simulink model "model_with_phases"  (R2018b)
settings: Solver=daessc  StartTime=0.0  StopTime=1  RelTol=1e-3
StopFcn:
  | % fault = 10
  | % location = 200
  | % fault_data
  | % simout=[simout,faults]
  | % simout(:,24) = location;
  | % data = xlsread('E:\testing data\test_data');
  | % data = [data;simout];
  | % xlswrite('E:\testing data\test_data',data);
libraries: powerlib x7, powerlib_meascontrol x2
settings Model: Creator=Edagotti Pavankumar  LastModifiedBy=Edagotti Pavankumar
settings SolverCC: ZeroCrossAlgorithm=Adaptive
settings DebuggingCC: IgnoredZcDiagnostic=none

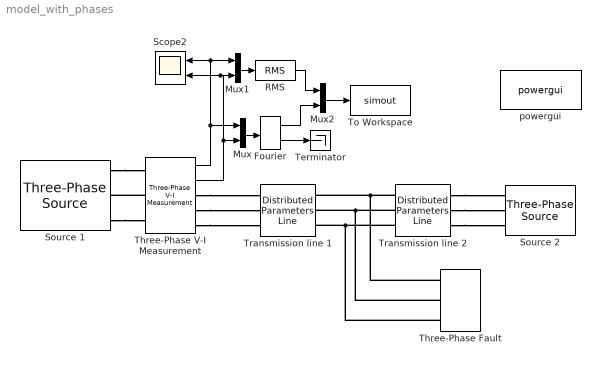
== system model_with_phases ==
  Fourier : powerlib_meascontrol/Measurements/Fourier  Freq=50  n=1  InInit=[0, 0]  Ts=0
      settings: SourceProductName=Simscape Power Systems
  Mux : Mux  Inputs=2
  Mux1 : Mux  Inputs=2
  Mux2 : Mux  Inputs=2
  RMS : powerlib_meascontrol/Measurements/RMS  TrueRMS=on  Freq=50  RMSInit=0  Ts=0
  Scope2 : Scope  NumInputPorts=2
  Source 1 : powerlib/Electrical Sources/Three-Phase Source  InternalConnection=Yg  VoltagePhases=off  Voltage=220e3  PhaseAngle=0  Voltage_phases=[25e3 25e3 25e3]/sqrt(3)  PhaseAngles_phases=[0 -120 +120]  Frequency=50  NonIdealSource=on  SpecifyImpedance=on  Resistance=0.8929  Inductance=16.58e-3  ShortCircuitLevel=100e6  BaseVoltage=220e3  XRratio=7  BusType=swing  Pref=10e3  Qref=0  Prefabc=[10e3, 10e3, 10e3]  Qrefabc=[0, 0, 0]  Qmin=-inf  Qmax=inf
  Source 2 : powerlib/Electrical Sources/Three-Phase Source  InternalConnection=Yg  VoltagePhases=off  Voltage=220e3  PhaseAngle=-40  Voltage_phases=[25e3 25e3 25e3]/sqrt(3)  PhaseAngles_phases=[0 -120 +120]  Frequency=50  NonIdealSource=on  SpecifyImpedance=on  Resistance=0.8929  Inductance=16.58e-3  ShortCircuitLevel=100e6  BaseVoltage=220e3  XRratio=7  BusType=PV  Pref=inf  Qref=0  Prefabc=[10e3, 10e3, 10e3]  Qrefabc=[0, 0, 0]  Qmin=-inf  Qmax=inf
  Terminator : Terminator
  Three-Phase V-I Measurement : powerlib/Measurements/Three-Phase V-I Measurement  VoltageMeasurement=phase-to-ground  SetLabelV=off  LabelV=Vabc  Vpu=on  VpuLL=off  CurrentMeasurement=yes  SetLabelI=off  LabelI=Iabc  Ipu=on  Pbase=100e6  Vbase=220e3  OutputType=Complex  PhasorSimulation=off  PSBequivalent=0
  Three-Phase Fault : powerlib/Elements/Three-Phase Fault  InitialStates=0  FaultA=on  FaultB=off  FaultC=off  GroundFault=on  SwitchTimes=0.5  External=off  SwitchStatus=NaN  FaultResistance=20  GroundResistance=0.001  SnubberResistance=1e6  SnubberCapacitance=inf  Measurements=None
  To Workspace : ToWorkspace  VariableName=simout  SampleTime=-1
      settings: MaxDataPoints=200  Save2DSignal=2-D array (concatenate along first dimension)
  Transmission line 1 : powerlib/Elements/Distributed Parameters Line  Phases=3  Frequency=50  Resistance=[0.0238 0.3885]  Inductance=[0.0009509508 0.0032508989]  Capacitance=[12.74e-9 7.751e-9]  Length=160  x1=[8.85875852267748e-10 256106.737010838 256106.73701084;314.159265358979 314.159265358979 314.159265358979;-0.991239322998321 -0.0183316743636767 -1.58912800115857]  x2=[8.93084897335148e-10 257720.727111479 257720.727111481;314.159265358979 314.159265358979 314.159265358979;-1.00602777839429 -0.045748220316972 -1.61654454711186]  x3=[1.76591819123062e-12 793.390665840204 793.390665840216;314.159265358979 314.159265358979 314.159265358979;-1.42146556624267 -0.176195220133282 -1.74699154692818]  x4=[1.53917367282649e-12 1076.93135796091 1076.93135796091;314.159265358979 314.159265358979 314.159265358979;-0.688414818704923 -0.0783802254355052 -1.6491765522304]  x5=0.000803157247848664  V1=[8.859e-10 2.561e+05 2.561e+05;314.2 314.2 314.2;-0.9912 -0.01833 -1.589]  V2=[8.931e-10 2.577e+05 2.577e+05;314.2 314.2 314.2;-1.006 -0.04575 -1.617]  I1=[1.766e-12 793.4 793.4;314.2 314.2 314.2;-1.421 -0.1762 -1.747]  I2=[1.539e-12 1077 1077;314.2 314.2 314.2;-0.6884 -0.07838 -1.649]  nHarmo=1  Measurements=None
      settings: SourceProductName=Simscape Power Systems
  Transmission line 2 : powerlib/Elements/Distributed Parameters Line  Phases=3  Frequency=50  Resistance=[0.0238 0.3885]  Inductance=[0.0009509508 0.0032508989]  Capacitance=[12.74e-9 7.751e-9]  Length=40  x1=[8.95741011278727e-10 257720.727111479 257720.727111481;314.159265358979 314.159265358979 314.159265358979;-0.814008885135909 0.085470215602079 -1.48532611119281]  x2=[8.89113759047248e-10 256920.332809656 256920.332809659;314.159265358979 314.159265358979 314.159265358979;-0.820988530494618 0.0790008961846263 -1.49179543061027]  x3=[2.24350221076048e-12 798.289373210214 798.289373210219;314.159265358979 314.159265358979 314.159265358979;-2.13671936046073 0.129729677301786 -1.44106664949311]  x4=[9.68167740404967e-13 1084.26106264654 1084.26106264656;314.159265358979 314.159265358979 314.159265358979;0.706934938878884 0.00929096905672002 -1.56150535773818]  x5=0.000200789311962166  V1=[8.957e-10 2.577e+05 2.577e+05;314.2 314.2 314.2;-0.814 0.08547 -1.485]  V2=[8.891e-10 2.569e+05 2.569e+05;314.2 314.2 314.2;-0.821 0.079 -1.492]  I1=[2.244e-12 798.3 798.3;314.2 314.2 314.2;-2.137 0.1297 -1.441]  I2=[9.682e-13 1084 1084;314.2 314.2 314.2;0.7069 0.009291 -1.562]  nHarmo=1  Measurements=None
      settings: SourceProductName=Simscape Power Systems
  powergui : powerlib/powergui  Priority=1  SimulationMode=Continuous  SampleTime=8.3333e-05  frequency=60  Iterations=50  frequencyindice=50  Pbase=100e6  ErrMax=1e-4  UnitsV=kV  UnitsW=MW  buscounter=0  FunctionMessages=off  echomessages=off  EnableUseOfTLC=off  CurrentSourceSwitches=off  DisableSnubberDevices=off  DisableRonSwitches=off  DisableVfSwitches=off  DisplayEquations=off  SolverType=Tustin/Backward Euler (TBE)  Interpol=off  ExternalGateDelay=off  methode=off  Ts=100  x0status=blocks  SPID=off  SwTol=0  HookPort=off  RestoreLinks=warning  ResistiveCurrentMeasurement=off  Frange=[0:2:500]  Ylog=off  Xlog=on  ShowGrid=off  save=off  variable=ZData  structure=0  ZoomFFT=off  StartTime=0.0  cycles=1  DisplayStyle=1  fundamental=60  FreqAxis=off  MaxFrequency=1000  frequencyindicesteady=1  RmsSteady=2  display=off
  wires:
  Fourier/1 -> Terminator/1
  Mux/1 -> Fourier/1
  Mux2/1 -> To Workspace/1
  Three-Phase V-I Measurement/2 -> Mux/2, Scope2/2, Mux1/2
  RMS/1 -> Mux2/1
  Three-Phase V-I Measurement/1 -> Mux/1, Mux1/1, Scope2/1
  Mux1/1 -> RMS/1
  Fourier/2 -> Mux2/2
  connections:
  Three-Phase V-I Measurement/RConn2 -- Transmission line 1/LConn2
  Three-Phase V-I Measurement/RConn1 -- Transmission line 1/LConn1
  Three-Phase V-I Measurement/RConn3 -- Transmission line 1/LConn3
  Source 1/RConn1 -- Three-Phase V-I Measurement/LConn1
  Transmission line 2/RConn1 -- Source 2/RConn1
  Transmission line 2/LConn2 -- Three-Phase Fault/LConn2 -- Transmission line 1/RConn2
  Transmission line 2/RConn2 -- Source 2/RConn2
  Source 1/RConn3 -- Three-Phase V-I Measurement/LConn3
  Transmission line 2/LConn3 -- Three-Phase Fault/LConn3 -- Transmission line 1/RConn3
  Three-Phase V-I Measurement/LConn2 -- Source 1/RConn2
  Transmission line 2/RConn3 -- Source 2/RConn3
  Transmission line 2/LConn1 -- Three-Phase Fault/LConn1 -- Transmission line 1/RConn1
